simulink model "chap13_1sim"  (Simulink 7.7)
settings: Solver=ode45  StartTime=0.0  StopTime=3  RelTol=1e-3
libraries: simulink x1
settings Model: Creator=Administrator  LastModifiedBy=ljk
settings CodeAppCC: CustomSymbolStrType=$N$R$M_T

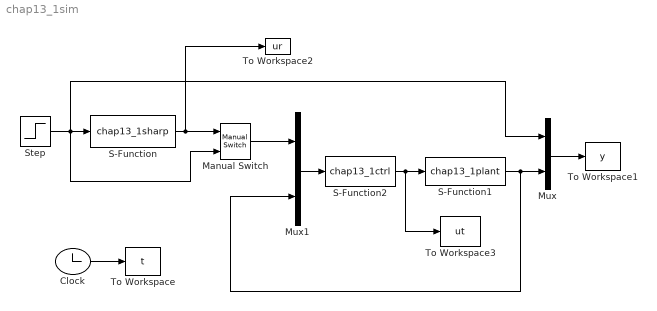
== system chap13_1sim ==
  Clock : Clock
      settings: Decimation=20
  Manual Switch : simulink/Signal Routing/Manual Switch  SystemSampleTime=-1  sw=1  action=0  varsize=off
  Mux : Mux  Inputs=2
  Mux1 : Mux  Inputs=2
  S-Function : S-Function  FunctionName=chap13_1sharp  EnableBusSupport=off
  S-Function1 : S-Function  FunctionName=chap13_1plant  EnableBusSupport=off
  S-Function2 : S-Function  FunctionName=chap13_1ctrl  EnableBusSupport=off
  Step : Step  Time=0  After=200  SampleTime=0
  To Workspace : ToWorkspace  VariableName=t  SampleTime=-1  SaveFormat=Array
  To Workspace1 : ToWorkspace  VariableName=y  SampleTime=-1  SaveFormat=Array
  To Workspace2 : ToWorkspace  VariableName=ur  SampleTime=-1  SaveFormat=Array
  To Workspace3 : ToWorkspace  VariableName=ut  SampleTime=-1  SaveFormat=Array
  wires:
  Step/1 -> S-Function/1, Mux/1, Manual Switch/2
  Mux/1 -> To Workspace1/1
  S-Function1/1 -> Mux/2, Mux1/2
  Clock/1 -> To Workspace/1
  S-Function2/1 -> S-Function1/1, To Workspace3/1
  Mux1/1 -> S-Function2/1
  Manual Switch/1 -> Mux1/1
  S-Function/1 -> To Workspace2/1, Manual Switch/1
